simulink model "case_15_maybe_crash"  (R2025b)
settings: Solver=VariableStepAuto  StartTime=0.0  StopTime=180  RelTol=1e-3
settings Model: Creator=sanborkl  LastModifiedBy=sanborkl

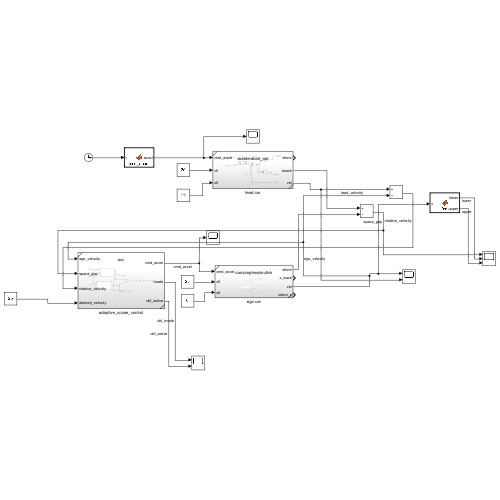
[thumbnail: Simulink's stored preview of the top-level diagram]
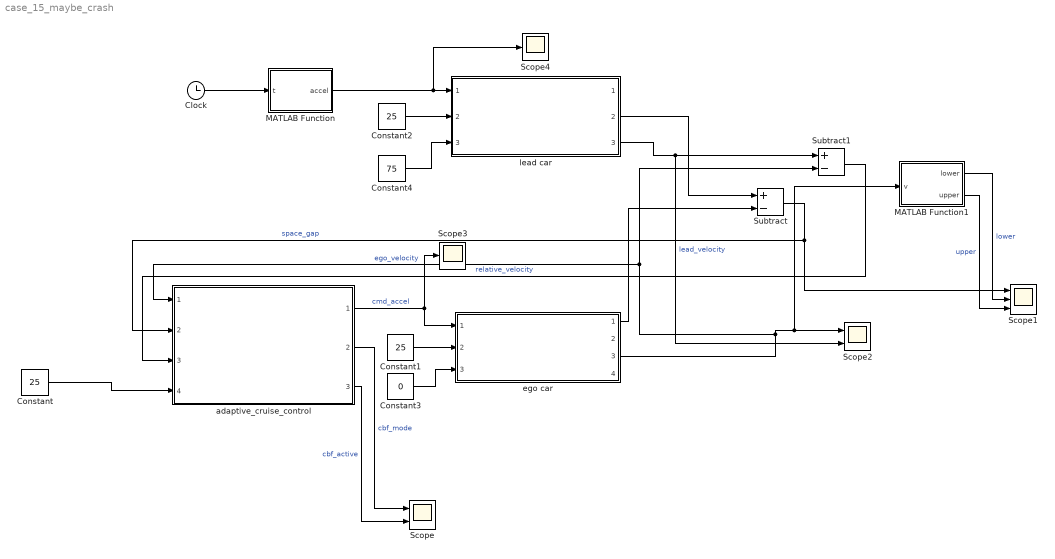
== system case_15_maybe_crash ==
  Clock : Clock
  Constant : Constant  Value=25
  Constant1 : Constant  Value=25
  Constant2 : Constant  Value=25
  Constant3 : Constant  Value=0
  Constant4 : Constant  Value=75
  MATLAB Function : MATLAB Function  TreatAsAtomicUnit=on
  MATLAB Function1 : MATLAB Function  TreatAsAtomicUnit=on
  Scope : Scope  NumInputPorts=2
      settings: ActiveDisplayYMinimum=0.90216044044736554  ActiveDisplayYMaximum=3.1697341365924903
  Scope1 : Scope  NumInputPorts=3
      settings: ActiveDisplayYMinimum=-0.22752940048412854  ActiveDisplayYMaximum=0.18107907358280398  YLabel=m
  Scope2 : Scope  NumInputPorts=2
      settings: ActiveDisplayYMinimum=-3.1249999999999991  ActiveDisplayYMaximum=28.125  YLabel=m/s  DataLoggingVariableName=ScopeData2
  Scope3 : Scope
      settings: ActiveDisplayYMinimum=-3.4073778564880728  ActiveDisplayYMaximum=0.666400708392654  YLabel=m/s^2  DataLoggingVariableName=ScopeData3
  Scope4 : Scope
      settings: ActiveDisplayYMinimum=-1  ActiveDisplayYMaximum=1  DataLoggingVariableName=ScopeData4
  Subtract : Sum  Inputs=+-
  Subtract1 : Sum  Inputs=+-
  adaptive_cruise_control : Subsystem  ReferencedSubsystem=acc
  ego car : Subsystem  ReferencedSubsystem=carcomplexsimulink
  lead car : Subsystem  ReferencedSubsystem=acceleration_car
  wires:
  ego car/3 -> Scope2/1, MATLAB Function1/1(v), Subtract1/2, adaptive_cruise_control/1  "ego_velocity"
  adaptive_cruise_control/1 -> ego car/1, Scope3/1  "cmd_accel"
  Constant1/1 -> ego car/2
  Subtract1/1 -> adaptive_cruise_control/3  "relative_velocity"
  lead car/3 -> Scope2/2, Subtract1/1  "lead_velocity"
  Constant3/1 -> ego car/3
  Constant2/1 -> lead car/2
  adaptive_cruise_control/2 -> Scope/1  "cbf_mode"
  lead car/2 -> Subtract/1
  adaptive_cruise_control/3 -> Scope/2  "cbf_active"
  Constant/1 -> adaptive_cruise_control/4
  ego car/1 -> Subtract/2
  Subtract/1 -> Scope1/1, adaptive_cruise_control/2  "space_gap"
  Constant4/1 -> lead car/3
  MATLAB Function/1(accel) -> Scope4/1, lead car/1
  MATLAB Function1/1(lower) -> Scope1/2  "lower"
  MATLAB Function1/2(upper) -> Scope1/3  "upper"
  Clock/1 -> MATLAB Function/1(t)

== matlab function case_15_maybe_crash/MATLAB Function ==
  data: t input; accel output
function accel = cmd_accel(t)

if t < 10.0
    accel = 0.0;
elseif t < 22.0
    accel = -2.0;
elseif t < 55.0
    accel = 0.0;
elseif t < 133.9
    accel = 0.2;
else
    accel = -5000;
end

== matlab function case_15_maybe_crash/MATLAB Function1 ==
  data: v input; lower output; upper output
function [lower, upper] = fcn(v)

lower = 2 * v + 5;
upper = 2 * v + 15;
